simulink model "lindiscrmodel_obs"  (R2019a)
settings: Solver=VariableStepAuto  StartTime=0.0  StopTime=30  RelTol=1e-3
InitFcn:
  | lindiscrmodel
values from neighbouring files (symbols this model uses):
  L1 = place(linmat.A1',linmat.C1',pdes1)'    [lindiscrmodel.m]
  Ts = 0.01    [lindiscrmodel.m]
undefined symbols (not defined in the file or in its folder): Discrete, linmat, Time
libraries: ctrlSharedLib x1
settings Model: Creator=jessi  LastModifiedBy=jessi

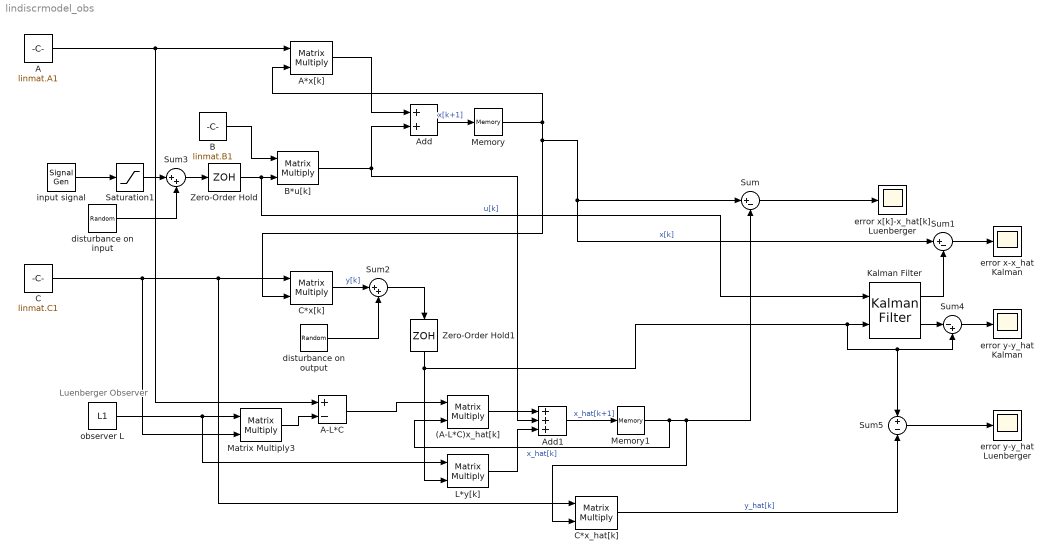
== system lindiscrmodel_obs ==
  note: Luenberger Observer
  (A-L*C)x_hat[k] : Product  Multiplication=Matrix(*)
  A : Constant  Value=linmat.A1  SampleTime=Ts
  A*x[k] : Product  Multiplication=Matrix(*)
  A-L*C : Sum  Inputs=+-
  Add : Sum
  Add1 : Sum  Inputs=+++
  B : Constant  Value=linmat.B1  SampleTime=Ts
  B*u[k] : Product  Multiplication=Matrix(*)
  C : Constant  Value=linmat.C1  SampleTime=Ts
  C*x[k] : Product  Multiplication=Matrix(*)
  C*x_hat[k] : Product  Multiplication=Matrix(*)
  Kalman Filter : ctrlSharedLib/Kalman Filter  TimeDomain=Discrete-Time  UseCurrentEstimator=on  ModelSource=Individual A, B, C, D matrices  ModelSourceVariable=sysd2  A=linmat.A1  B=linmat.B1  C=linmat.C1  D=linmat.D1  NumberOfStates=1  NumberOfInputs=1  NumberOfOutputs=1  InitialEstimateSource=Dialog  X0=[0;0;0;0]  P0=10  UseK=off  UseGH=off  NumberOfProcessNoiseInputs=1  G=1  TimeInvariantG=on  H=0  TimeInvariantH=on  Q=diag([100 100 0.01 0.01])  TimeInvariantQ=on  R=0.0001  TimeInvariantR=on  N=0  TimeInvariantN=on  AddInputPort=on  AddEnablePort=off  OutputEstimatedY=on  OutputP=off  Ts=Ts
      settings: SourceProductBaseCode=CT
  L*y[k] : Product  Multiplication=Matrix(*)
  Matrix Multiply3 : Product  Multiplication=Matrix(*)
  Memory : Memory  InitialCondition=[0;0;0;0]
  Memory1 : Memory  InitialCondition=[0;0;0;0]
  Saturation1 : Saturate  UpperLimit=1  LowerLimit=-1
  Sum : Sum  Inputs=|+-
  Sum1 : Sum  Inputs=|+-
  Sum2 : Sum  Inputs=|++
  Sum3 : Sum  Inputs=|++
  Sum4 : Sum  Inputs=|-+
  Sum5 : Sum  Inputs=+-
  Zero-Order Hold : ZeroOrderHold  SampleTime=Ts
  Zero-Order Hold1 : ZeroOrderHold  SampleTime=Ts
  disturbance on input : RandomNumber  Variance=0  SampleTime=0.1
  disturbance on output : RandomNumber  Variance=0.1  SampleTime=0.1
  error x-x_hat Kalman : Scope
  error x[k]-x_hat[k] Luenberger : Scope
  error y-y_hat Kalman : Scope
  error y-y_hat Luenberger : Scope
  input signal : SignalGenerator  WaveForm=square  Amplitude=0
  observer L : Constant  Value=L1  SampleTime=Ts
  wires:
  input signal/1 -> Saturation1/1
  B/1 -> B*u[k]/1
  A/1 -> A-L*C/1, A*x[k]/1
  A*x[k]/1 -> Add/1
  B*u[k]/1 -> Add1/2, Add/2
  Memory/1 -> A*x[k]/2, Sum/1, Sum1/1, C*x[k]/2  "x[k]"
  C/1 -> Matrix Multiply3/2, C*x_hat[k]/1, C*x[k]/1
  observer L/1 -> L*y[k]/1, Matrix Multiply3/1
  Matrix Multiply3/1 -> A-L*C/2
  A-L*C/1 -> (A-L*C)x_hat[k]/1
  (A-L*C)x_hat[k]/1 -> Add1/1
  L*y[k]/1 -> Add1/3
  Add1/1 -> Memory1/1  "x_hat[k+1]"
  Memory1/1 -> C*x_hat[k]/2, Sum/2, (A-L*C)x_hat[k]/2  "x_hat[k]"
  Add/1 -> Memory/1  "x[k+1]"
  Sum/1 -> error x[k]-x_hat[k] Luenberger/1
  Sum1/1 -> error x-x_hat Kalman/1
  Kalman Filter/1 -> Sum1/2
  Sum3/1 -> Zero-Order Hold/1
  Saturation1/1 -> Sum3/1
  Zero-Order Hold/1 -> Kalman Filter/1, B*u[k]/2  "u[k]"
  disturbance on input/1 -> Sum3/2
  C*x[k]/1 -> Sum2/1  "y[k]"
  disturbance on output/1 -> Sum2/2
  Kalman Filter/2 -> Sum4/1
  Sum4/1 -> error y-y_hat Kalman/1
  Sum2/1 -> Zero-Order Hold1/1
  Sum5/1 -> error y-y_hat Luenberger/1
  C*x_hat[k]/1 -> Sum5/2  "y_hat[k]"
  Zero-Order Hold1/1 -> Kalman Filter/2, Sum5/1, Sum4/2, L*y[k]/2
